simulink model "AtrasoAdelanto"  (R2017b)
settings: Solver=VariableStepAuto  StartTime=0.0  StopTime=50  RelTol=1e-3
libraries: simulink x1
settings Model: Creator=Cx001la  LastModifiedBy=Cx001la

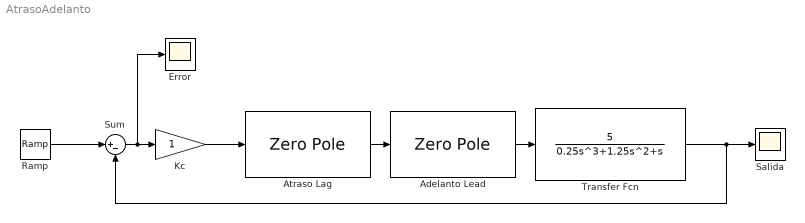
== system AtrasoAdelanto ==
  Adelanto Lead : ZeroPole  Zeros=[-0.495]  Poles=[-5.51]
  Atraso Lag : ZeroPole  Zeros=[-0.2]  Poles=[-0.009832]
  Error : Scope
  Kc : Gain
  Ramp : simulink/Sources/Ramp  slope=1  start=0  X0=0
  Salida : Scope
  Sum : Sum  Inputs=|+-
  Transfer Fcn : TransferFcn  Numerator=[5]  Denominator=[0.25 1.25 1 0]
  wires:
  Ramp/1 -> Sum/1
  Sum/1 -> Error/1, Kc/1
  Atraso Lag/1 -> Adelanto Lead/1
  Kc/1 -> Atraso Lag/1
  Adelanto Lead/1 -> Transfer Fcn/1
  Transfer Fcn/1 -> Sum/2, Salida/1
